simulink model "CRC_Test_2"  (R2019a)
settings: Solver=VariableStepAuto  StartTime=0.0  StopTime=7  RelTol=1e-3
values from neighbouring files (symbols this model uses):
  data_length = length(data)    [CRC_Generator.m]    (also in matlab.mat = 10)
  generate_polynomial = [1 0 1 1]    [matlab.mat]
libraries: commcrc2 x2, dspsrcs4 x1, dspsigops x1, commutil2 x1
settings Model: Creator=kaili  LastModifiedBy=kaili
settings SFSimCC: SimParseCustomCode=off
settings GRTTargetCC: CombineOutputUpdateFcns=off  MatFileLogging=off
settings ConfigComp: PLC_TargetIDE=codesys35  PLC_GenerateReport=off  PLC_LaunchReport=off

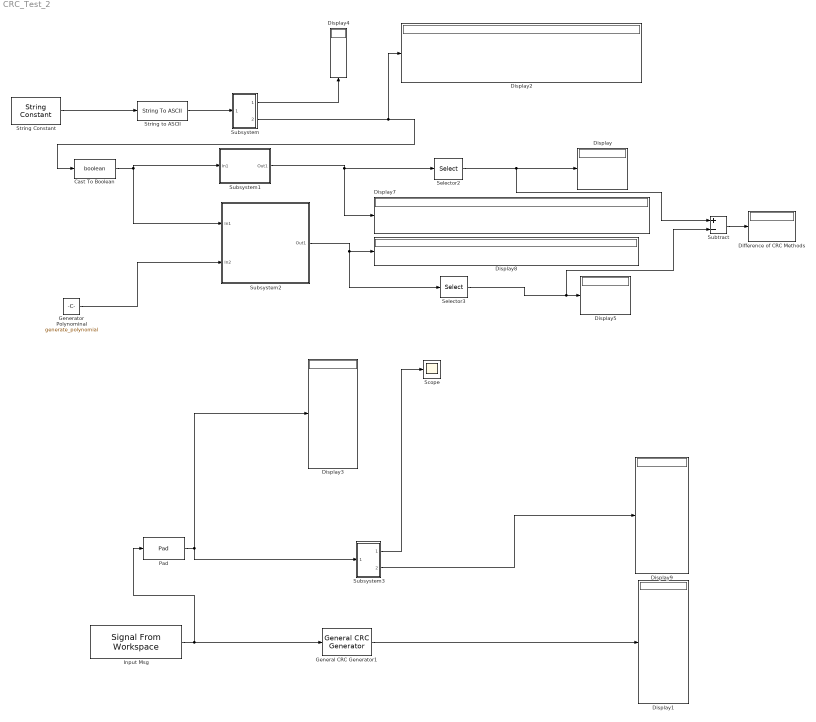
== system CRC_Test_2 ==
  Cast To Boolean : DataTypeConversion  OutDataTypeStr=boolean
  Difference of CRC Methods : Display
  Display{,1..5,7..9} (9 alike) : Display
  General CRC Generator1 : commcrc2/General CRC Generator  genPoly=[1 0 1 1]  iniStates=[0]  directMethod=off  reflectInputBytes=off  reflectChecksums=off  finalXOR=0  numChecksums=1
      settings: SourceProductName=Communications Toolbox  SourceProductBaseCode=CM
  Generator Polynominal : Constant  Value=generate_polynomial
  "Input Msg " : dspsrcs4/Signal From Workspace  X=[1 0 1 1 1 1 1 0]  Ts=1  nsamps=8  OutputAfterFinalValue=Cyclic repetition  ignoreOrWarnInputAndFrameLengths=off  OutputFrames=off
  Pad : dspsigops/Pad  padAlong=Columns  dimsToPad=1  valSrc=Specify via dialog  padVal=0  spec=Output size  padNumOutRowsSpecMethod=User-specified  numOutRows=11  padNumOutColsSpecMethod=User-specified  numOutCols=3  isVarDimsMode=off  padBeginning=0  padEnd=0  outSizeMode=User-specified  outSize=1  padSigAt=End  trunc_flag=None  roundingMode=Floor  overflowMode=off  truncOrWrapMode=Truncate  wrap_flag=None
      settings: SourceProductName=DSP System Toolbox  SourceProductBaseCode=DS
  Scope : Scope
  Selector2 : Selector  InputPortWidth=data_length+3  IndexOptions=Index vector (dialog)  Indices=[data_length+1:data_length+3]  OutputSizes=1
  Selector3 : Selector  InputPortWidth=10+3  IndexOptions=Index vector (dialog)  Indices=[data_length+1:data_length+3]  OutputSizes=1
  String Constant : StringConstant  String="\"HKL\""
  String to ASCII : StringToASCII
  Subsystem : Subsystem  TreatAsAtomicUnit=on
  Subsystem1 : Subsystem  TreatAsAtomicUnit=on
  Subsystem2 : Subsystem  TreatAsAtomicUnit=on
  Subsystem3 : Subsystem  TreatAsAtomicUnit=on
  Subtract : Sum  Inputs=+-
  wires:
  Selector2/1 -> Subtract/1, Display/1
  General CRC Generator1/1 -> Display1/1
  Selector3/1 -> Subtract/2, Display5/1
  "Input Msg "/1 -> Pad/1, General CRC Generator1/1
  Generator Polynominal/1 -> Subsystem2/2(In2)
  Subsystem/2(Out2) -> Cast To Boolean/1, Display2/1
  Subsystem/1(Out1) -> Display4/1
  Subsystem1/1(Out1) -> Display7/1, Selector2/1
  Subsystem2/1(Out1) -> Selector3/1, Display8/1
  Cast To Boolean/1 -> Subsystem2/1(In1), Subsystem1/1(In1)
  String Constant/1 -> String to ASCII/1
  String to ASCII/1 -> Subsystem/1(Input)
  Subtract/1 -> Difference of CRC Methods/1
  Pad/1 -> Subsystem3/1(In1), Display3/1
  Subsystem3/1(Out1) -> Scope/1
  Subsystem3/2(Out2) -> Display9/1

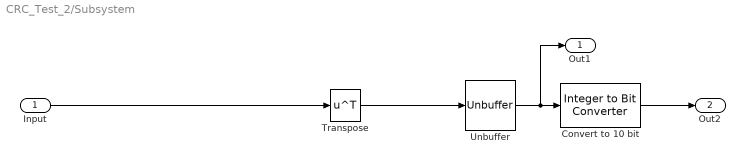
== system CRC_Test_2/Subsystem ==
  Input : Inport
  Convert to 10 bit : commutil2/Integer to Bit Converter  nbits=10  signedInputValues=Unsigned  bitOrder=MSB first  outDtype=Inherit via internal rule
      settings: SourceProductName=Communications Toolbox
  Transpose : Math  Operator=transpose  SaturateOnIntegerOverflow=on
  Unbuffer : Unbuffer
  Out1 : Outport
  Out2 : Outport  Port=2
  wires:
  Input/1 -> Transpose/1
  Convert to 10 bit/1 -> Out2/1
  Transpose/1 -> Unbuffer/1
  Unbuffer/1 -> Out1/1, Convert to 10 bit/1

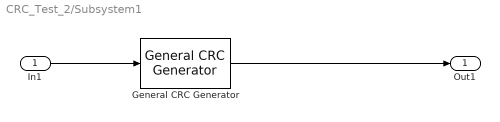
== system CRC_Test_2/Subsystem1 ==
  In1 : Inport
  General CRC Generator : commcrc2/General CRC Generator  genPoly=generate_polynomial  iniStates=[ 0 ]  directMethod=off  reflectInputBytes=off  reflectChecksums=off  finalXOR=0  numChecksums=1
      settings: SourceProductName=Communications Toolbox  SourceProductBaseCode=CM
  Out1 : Outport
  wires:
  General CRC Generator/1 -> Out1/1
  In1/1 -> General CRC Generator/1

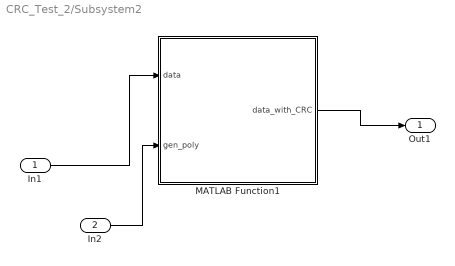
== system CRC_Test_2/Subsystem2 ==
  In1 : Inport
  In2 : Inport  Port=2
  MATLAB Function1 : MATLAB Function  TreatAsAtomicUnit=on
  Out1 : Outport
  wires:
  In2/1 -> MATLAB Function1/2(gen_poly)
  MATLAB Function1/1(data_with_CRC) -> Out1/1
  In1/1 -> MATLAB Function1/1(data)

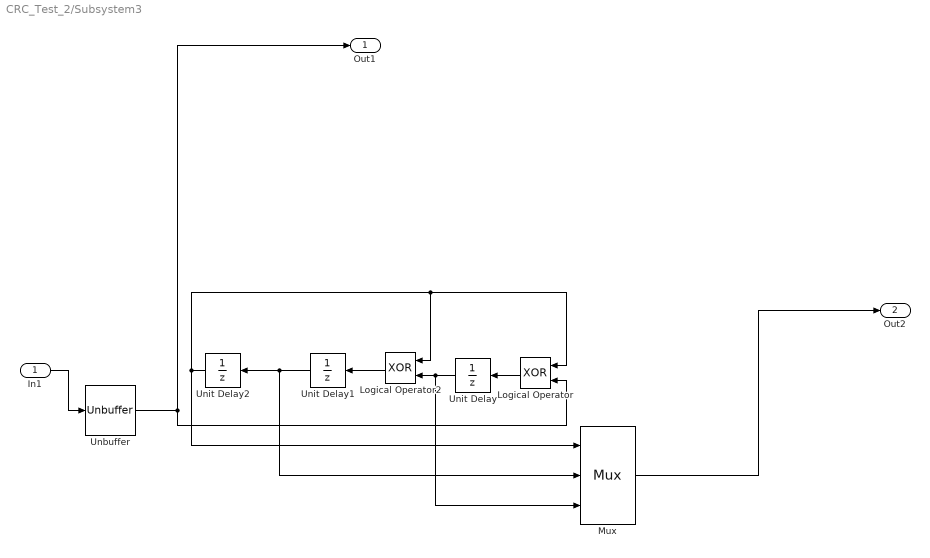
== system CRC_Test_2/Subsystem3 ==
  In1 : Inport
  Logical Operator : Logic  Operator=XOR  AllPortsSameDT=off  OutDataTypeStr=boolean
  Logical Operator2 : Logic  Operator=XOR  AllPortsSameDT=off  OutDataTypeStr=boolean
  Mux : Mux  Inputs=3
  Unbuffer : Unbuffer
  Unit Delay : UnitDelay  SampleTime=-1  HasFrameUpgradeWarning=on
  Unit Delay1 : UnitDelay  SampleTime=-1  HasFrameUpgradeWarning=on
  Unit Delay2 : UnitDelay  SampleTime=-1  HasFrameUpgradeWarning=on
  Out1 : Outport
  Out2 : Outport  Port=2
  wires:
  Unbuffer/1 -> Out1/1, Logical Operator/2
  Unit Delay2/1 -> Mux/1, Logical Operator2/1, Logical Operator/1
  Unit Delay/1 -> Mux/3, Logical Operator2/2
  Unit Delay1/1 -> Mux/2, Unit Delay2/1
  Logical Operator2/1 -> Unit Delay1/1
  Logical Operator/1 -> Unit Delay/1
  Mux/1 -> Out2/1
  In1/1 -> Unbuffer/1

== matlab function CRC_Test_2/Subsystem2/MATLAB Function1 ==
  data: data input; data_with_CRC output; gen_poly input
%data: row vector of logical 1 and 0 bits
% gen_poly: row vector  representing the polynom

function data_with_CRC = CRC_Generator(data,gen_poly)
data_length=length(data);
CRC_length = length(gen_poly)-1;
CRC_Code = zeros(CRC_length,1);
index = 1;
zrs = zeros(CRC_length+1,1);
data_append=[logical(data); zrs];
current_data = data_append(index:CRC_length+index);
tmp=zeros(CRC_length+1,1);
tmp_index=1;
data_start=0;
to_add = 0;
while index <= data_length
    tmp = bitxor(current_data,gen_poly);
    [k r] = max( tmp~=0, [], 1 ); %k max in row, r index of max
    if k~=0
%         coder.varsize('tt');
% %         tt=find(tmp~=0,1);
%         tt=strfind(tmp,[0 1]);
%         tmp_index = tt(1);
        tmp_index = r(1);
    else
        tmp_index=CRC_length+2;
    end
    data_start = index+CRC_length+1;
    prev_index = index;
    index = index + tmp_index-1;
    to_add = tmp_index-1;
    %find a way to do this using fixed size arrays to make PLC successful
    if index > data_length
        tmp_curr = tmp(data_length-prev_index+2:end);
        current_data_ = [tmp_curr;false(1,CRC_length+1-length(tmp_curr))'];
        current_data = current_data_(1:CRC_length+1,1);
        break;
    else
        current_data_ = [tmp(tmp_index:end); data_append(data_start:data_start+to_add-1)];
        current_data = current_data_(1:CRC_length+1,1);
    end
end

CRC_Code = current_data(1:CRC_length);



data_with_CRC = logical([data; CRC_Code]);
